simulink model "validazione_modello"  (R2021a)
settings: Solver=FixedStepAuto  StartTime=0.0  StopTime=10.0  FixedStep=Tc  RelTol=1e-3
values from neighbouring files (symbols this model uses):
  a1 = a(2)    [esercizio2.m]
  a2 = a(3)    [esercizio2.m]
  a3 = a(4)    [esercizio2.m]
  a4 = a(5)    [esercizio2.m]
  b0 = b(1)    [esercizio2.m]
  b1 = b(2)    [esercizio2.m]
  b2 = b(3)    [esercizio2.m]
  b3 = b(4)    [esercizio2.m]
  b4 = b(5)    [esercizio2.m]
settings Model: Creator=Giorgio  LastModifiedBy=Giorgio

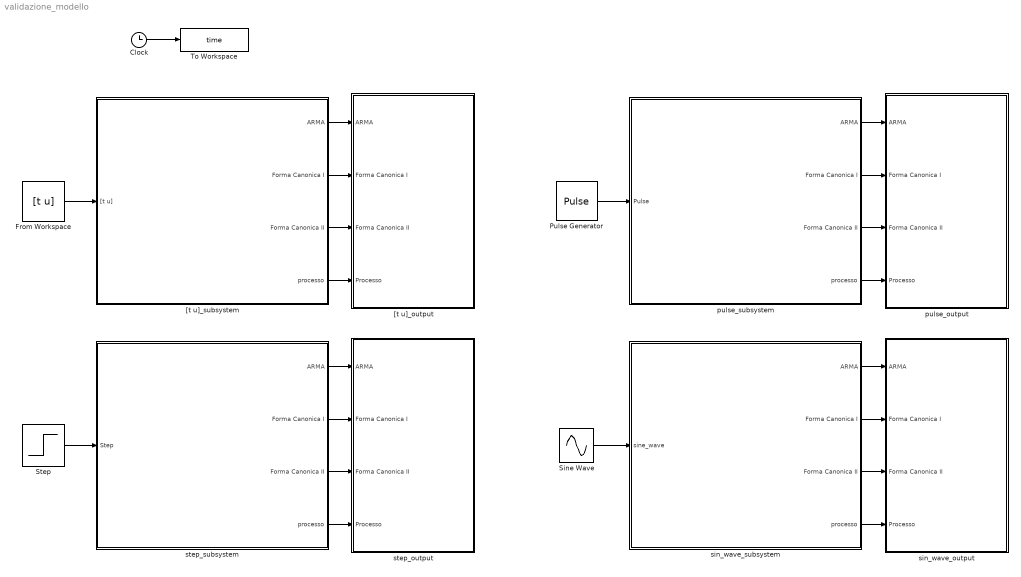
== system validazione_modello ==
  Clock : Clock
  From Workspace : FromWorkspace  VariableName=[t u]
  Pulse Generator : DiscretePulseGenerator  PulseType=Time based  Period=1  PulseWidth=50
  Sine Wave : Sin  Amplitude=0.5  Frequency=4  SampleTime=0
  Step : Step  Time=0  SampleTime=0
  To Workspace : ToWorkspace  VariableName=time  SampleTime=-1
      settings: Save2DSignal=2-D array (concatenate along first dimension)
  "[t u]_output" : Subsystem
  "[t u]_subsystem" : Subsystem
  pulse_output : Subsystem
  pulse_subsystem : Subsystem
  sin_wave_output : Subsystem
  sin_wave_subsystem : Subsystem
  step_output : Subsystem
  step_subsystem : Subsystem
  wires:
  From Workspace/1 -> "[t u]_subsystem"/1("[t u]")
  "[t u]_subsystem"/1(ARMA) -> "[t u]_output"/1(ARMA)
  "[t u]_subsystem"/2(Forma Canonica I) -> "[t u]_output"/2(Forma Canonica I)
  "[t u]_subsystem"/3(Forma Canonica II) -> "[t u]_output"/3(Forma Canonica II)
  "[t u]_subsystem"/4(processo) -> "[t u]_output"/4(Processo)
  step_subsystem/3(Forma Canonica II) -> step_output/3(Forma Canonica II)
  step_subsystem/4(processo) -> step_output/4(Processo)
  Step/1 -> step_subsystem/1(Step)
  step_subsystem/2(Forma Canonica I) -> step_output/2(Forma Canonica I)
  step_subsystem/1(ARMA) -> step_output/1(ARMA)
  pulse_subsystem/1(ARMA) -> pulse_output/1(ARMA)
  pulse_subsystem/3(Forma Canonica II) -> pulse_output/3(Forma Canonica II)
  pulse_subsystem/4(processo) -> pulse_output/4(Processo)
  pulse_subsystem/2(Forma Canonica I) -> pulse_output/2(Forma Canonica I)
  Pulse Generator/1 -> pulse_subsystem/1(Pulse)
  Clock/1 -> To Workspace/1
  sin_wave_subsystem/3(Forma Canonica II) -> sin_wave_output/3(Forma Canonica II)
  Sine Wave/1 -> sin_wave_subsystem/1(sine_wave)
  sin_wave_subsystem/2(Forma Canonica I) -> sin_wave_output/2(Forma Canonica I)
  sin_wave_subsystem/4(processo) -> sin_wave_output/4(Processo)
  sin_wave_subsystem/1(ARMA) -> sin_wave_output/1(ARMA)

== system validazione_modello/[t u]_output ==
  ARMA : Inport
  Forma Canonica I : Inport  Port=2
  Forma Canonica II : Inport  Port=3
  Processo : Inport  Port=4
  Mux : Mux
  To Workspace12 : ToWorkspace  VariableName=tu_output  SampleTime=-1
      settings: Save2DSignal=2-D array (concatenate along first dimension)
  wires:
  Mux/1 -> To Workspace12/1
  Processo/1 -> Mux/4
  Forma Canonica II/1 -> Mux/3
  ARMA/1 -> Mux/1
  Forma Canonica I/1 -> Mux/2

== system validazione_modello/[t u]_subsystem ==
  "[t u]" : Inport
  Forma Canonica di tipo I : Subsystem
  Forma Canonica di tipo II : Subsystem
  Processo : MATLABSystem  System=linSysObj  SimulateUsing=Interpreted execution
      mask Type: linSysObj
      mask Display:
      | disp('Black box');
      | port_label('input',1,'u');
      | port_label('output',1,'y');
  modello ARMA : Subsystem
  ARMA : Outport
  Forma Canonica I : Outport  Port=2
  Forma Canonica II : Outport  Port=3
  processo : Outport  Port=4
  wires:
  "[t u]"/1 -> Processo/1, Forma Canonica di tipo II/1(u(k)), Forma Canonica di tipo I/1(u(k)), modello ARMA/1(u(k))
  modello ARMA/1(y(k)) -> ARMA/1
  Forma Canonica di tipo I/1(y(k)) -> Forma Canonica I/1
  Forma Canonica di tipo II/1(y(k)) -> Forma Canonica II/1
  Processo/1 -> processo/1

== system validazione_modello/pulse_output ==
  ARMA : Inport
  Forma Canonica I : Inport  Port=2
  Forma Canonica II : Inport  Port=3
  Processo : Inport  Port=4
  Mux : Mux
  To Workspace : ToWorkspace  VariableName=pulse_processo  SampleTime=-1
      settings: Save2DSignal=2-D array (concatenate along first dimension)
  To Workspace1 : ToWorkspace  VariableName=pulse_ARMA  SampleTime=-1
      settings: Save2DSignal=2-D array (concatenate along first dimension)
  To Workspace12 : ToWorkspace  VariableName=pulse_output  SampleTime=-1
      settings: Save2DSignal=2-D array (concatenate along first dimension)
  wires:
  Mux/1 -> To Workspace12/1
  Processo/1 -> To Workspace/1, Mux/4
  Forma Canonica II/1 -> Mux/3
  ARMA/1 -> To Workspace1/1, Mux/1
  Forma Canonica I/1 -> Mux/2

== system validazione_modello/pulse_subsystem ==
  Pulse : Inport
  Forma Canonica di tipo I : Subsystem
  Forma Canonica di tipo II : Subsystem
  Processo : MATLABSystem  System=linSysObj  SimulateUsing=Interpreted execution
      mask Type: linSysObj
      mask Display:
      | disp('Black box');
      | port_label('input',1,'u');
      | port_label('output',1,'y');
  modello ARMA : Subsystem
  ARMA : Outport
  Forma Canonica I : Outport  Port=2
  Forma Canonica II : Outport  Port=3
  processo : Outport  Port=4
  wires:
  Pulse/1 -> Processo/1, Forma Canonica di tipo II/1(u(k)), Forma Canonica di tipo I/1(u(k)), modello ARMA/1(u(k))
  modello ARMA/1(y(k)) -> ARMA/1
  Forma Canonica di tipo I/1(y(k)) -> Forma Canonica I/1
  Forma Canonica di tipo II/1(y(k)) -> Forma Canonica II/1
  Processo/1 -> processo/1

== system validazione_modello/sin_wave_output ==
  ARMA : Inport
  Forma Canonica I : Inport  Port=2
  Forma Canonica II : Inport  Port=3
  Processo : Inport  Port=4
  Mux : Mux
  To Workspace : ToWorkspace  VariableName=sine_wave_ARMA  SampleTime=-1
      settings: Save2DSignal=2-D array (concatenate along first dimension)
  To Workspace1 : ToWorkspace  VariableName=sine_wave_processo  SampleTime=-1
      settings: Save2DSignal=2-D array (concatenate along first dimension)
  To Workspace12 : ToWorkspace  VariableName=sine_wave_output  SampleTime=-1
      settings: Save2DSignal=2-D array (concatenate along first dimension)
  wires:
  Mux/1 -> To Workspace12/1
  Processo/1 -> To Workspace1/1, Mux/4
  Forma Canonica II/1 -> Mux/3
  ARMA/1 -> To Workspace/1, Mux/1
  Forma Canonica I/1 -> Mux/2

== system validazione_modello/sin_wave_subsystem ==
  sine_wave : Inport
  Forma Canonica di tipo I : Subsystem
  Forma Canonica di tipo II : Subsystem
  Processo : MATLABSystem  System=linSysObj  SimulateUsing=Interpreted execution
      mask Type: linSysObj
      mask Display:
      | disp('Black box');
      | port_label('input',1,'u');
      | port_label('output',1,'y');
  modello ARMA : Subsystem
  ARMA : Outport
  Forma Canonica I : Outport  Port=2
  Forma Canonica II : Outport  Port=3
  processo : Outport  Port=4
  wires:
  sine_wave/1 -> Processo/1, Forma Canonica di tipo II/1(u(k)), Forma Canonica di tipo I/1(u(k)), modello ARMA/1(u(k))
  modello ARMA/1(y(k)) -> ARMA/1
  Forma Canonica di tipo I/1(y(k)) -> Forma Canonica I/1
  Forma Canonica di tipo II/1(y(k)) -> Forma Canonica II/1
  Processo/1 -> processo/1

== system validazione_modello/step_output ==
  ARMA : Inport
  Forma Canonica I : Inport  Port=2
  Forma Canonica II : Inport  Port=3
  Processo : Inport  Port=4
  Mux : Mux
  To Workspace : ToWorkspace  VariableName=step_processo  SampleTime=-1
      settings: Save2DSignal=2-D array (concatenate along first dimension)
  To Workspace1 : ToWorkspace  VariableName=step_ARMA  SampleTime=-1
      settings: Save2DSignal=2-D array (concatenate along first dimension)
  To Workspace12 : ToWorkspace  VariableName=step_output  SampleTime=-1
      settings: Save2DSignal=2-D array (concatenate along first dimension)
  wires:
  Mux/1 -> To Workspace12/1
  Processo/1 -> Mux/4, To Workspace/1
  Forma Canonica II/1 -> Mux/3
  ARMA/1 -> Mux/1, To Workspace1/1
  Forma Canonica I/1 -> Mux/2

== system validazione_modello/step_subsystem ==
  Step : Inport
  Forma Canonica di tipo I : Subsystem
  Forma Canonica di tipo II : Subsystem
  Processo : MATLABSystem  System=linSysObj  SimulateUsing=Interpreted execution
      mask Type: linSysObj
      mask Display:
      | disp('Black box');
      | port_label('input',1,'u');
      | port_label('output',1,'y');
  modello ARMA : Subsystem
  ARMA : Outport
  Forma Canonica I : Outport  Port=2
  Forma Canonica II : Outport  Port=3
  processo : Outport  Port=4
  wires:
  Step/1 -> Processo/1, Forma Canonica di tipo II/1(u(k)), Forma Canonica di tipo I/1(u(k)), modello ARMA/1(u(k))
  modello ARMA/1(y(k)) -> ARMA/1
  Forma Canonica di tipo I/1(y(k)) -> Forma Canonica I/1
  Forma Canonica di tipo II/1(y(k)) -> Forma Canonica II/1
  Processo/1 -> processo/1

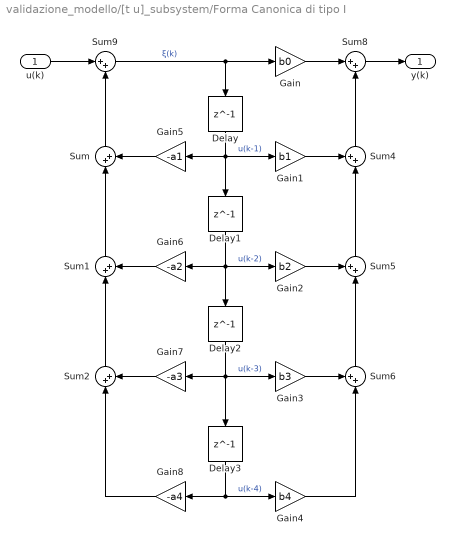
== system validazione_modello/[t u]_subsystem/Forma Canonica di tipo I ==
  u(k) : Inport
  Delay{,1..3} (4 alike) : Delay  DelayLength=1
  Gain : Gain  Gain=b0
  Gain1 : Gain  Gain=b1
  Gain2 : Gain  Gain=b2
  Gain3 : Gain  Gain=b3
  Gain4 : Gain  Gain=b4
  Gain5 : Gain  Gain=-a1
  Gain6 : Gain  Gain=-a2
  Gain7 : Gain  Gain=-a3
  Gain8 : Gain  Gain=-a4
  Sum{,1..2,8..9} (5 alike) : Sum  Inputs=|++
  Sum4 : Sum  Inputs=++|
  Sum5 : Sum  Inputs=++|
  Sum6 : Sum  Inputs=++|
  y(k) : Outport
  wires:
  Sum1/1 -> Sum/1
  Sum2/1 -> Sum1/1
  Gain8/1 -> Sum2/1
  Sum8/1 -> y(k)/1
  Sum4/1 -> Sum8/2
  Sum5/1 -> Sum4/2
  Sum6/1 -> Sum5/2
  Gain4/1 -> Sum6/2
  Delay/1 -> Gain1/1, Delay1/1, Gain5/1  "u(k-1)"
  Delay1/1 -> Delay2/1, Gain6/1, Gain2/1  "u(k-2)"
  Delay2/1 -> Gain7/1, Gain3/1, Delay3/1  "u(k-3)"
  Delay3/1 -> Gain8/1, Gain4/1  "u(k-4)"
  Sum/1 -> Sum9/2
  u(k)/1 -> Sum9/1
  Sum9/1 -> Gain/1, Delay/1  "ξ(k)"
  Gain/1 -> Sum8/1
  Gain1/1 -> Sum4/1
  Gain2/1 -> Sum5/1
  Gain3/1 -> Sum6/1
  Gain5/1 -> Sum/2
  Gain6/1 -> Sum1/2
  Gain7/1 -> Sum2/2

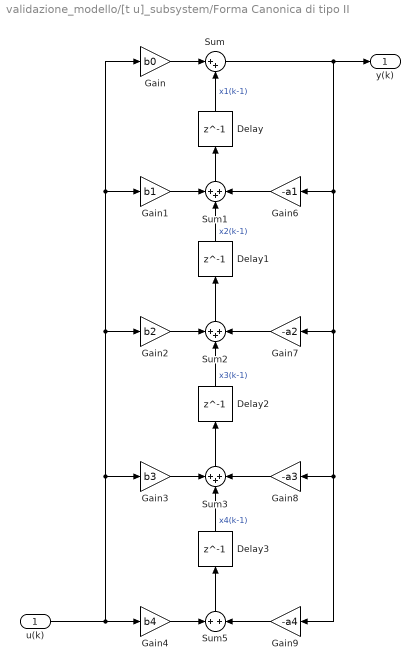
== system validazione_modello/[t u]_subsystem/Forma Canonica di tipo II ==
  u(k) : Inport
  Delay{,1..3} (4 alike) : Delay  DelayLength=1
  Gain : Gain  Gain=b0
  Gain1 : Gain  Gain=b1
  Gain2 : Gain  Gain=b2
  Gain3 : Gain  Gain=b3
  Gain4 : Gain  Gain=b4
  Gain6 : Gain  Gain=-a1
  Gain7 : Gain  Gain=-a2
  Gain8 : Gain  Gain=-a3
  Gain9 : Gain  Gain=-a4
  Sum : Sum  Inputs=|++
  Sum1 : Sum  Inputs=+++
  Sum2 : Sum  Inputs=+++
  Sum3 : Sum  Inputs=+++
  Sum5 : Sum  Inputs=+|+
  y(k) : Outport
  wires:
  u(k)/1 -> Gain4/1, Gain3/1, Gain2/1, Gain/1, Gain1/1
  Sum/1 -> Gain6/1, Gain7/1, Gain8/1, Gain9/1, y(k)/1
  Gain/1 -> Sum/1
  Sum1/1 -> Delay/1
  Sum2/1 -> Delay1/1
  Sum3/1 -> Delay2/1
  Gain1/1 -> Sum1/1
  Gain2/1 -> Sum2/1
  Gain3/1 -> Sum3/1
  Gain4/1 -> Sum5/1
  Gain8/1 -> Sum3/3
  Gain7/1 -> Sum2/3
  Gain6/1 -> Sum1/3
  Gain9/1 -> Sum5/2
  Delay/1 -> Sum/2  "x1(k-1)"
  Delay1/1 -> Sum1/2  "x2(k-1)"
  Delay2/1 -> Sum2/2  "x3(k-1)"
  Sum5/1 -> Delay3/1
  Delay3/1 -> Sum3/2  "x4(k-1)"

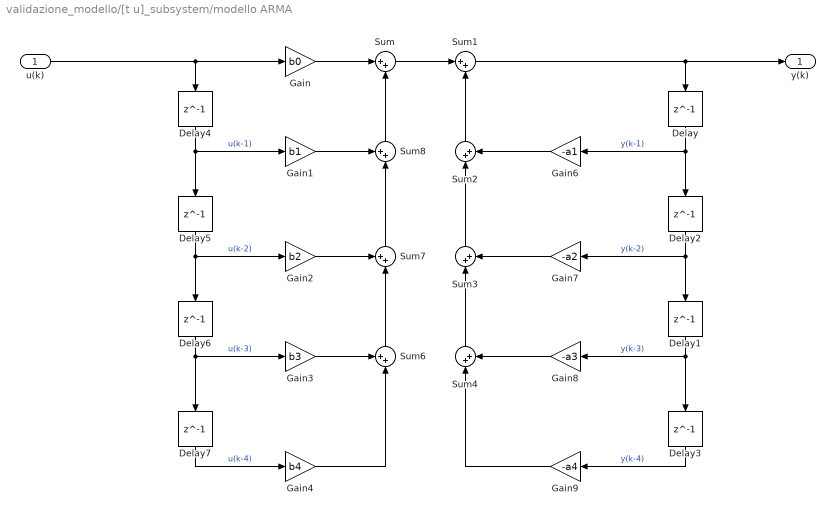
== system validazione_modello/[t u]_subsystem/modello ARMA ==
  u(k) : Inport
  Delay{,1..7} (8 alike) : Delay  DelayLength=1
  Gain : Gain  Gain=b0
  Gain1 : Gain  Gain=b1
  Gain2 : Gain  Gain=b2
  Gain3 : Gain  Gain=b3
  Gain4 : Gain  Gain=b4
  Gain6 : Gain  Gain=-a1
  Gain7 : Gain  Gain=-a2
  Gain8 : Gain  Gain=-a3
  Gain9 : Gain  Gain=-a4
  Sum{,1..4} (5 alike) : Sum  Inputs=|++
  Sum6 : Sum  Inputs=++|
  Sum7 : Sum  Inputs=++|
  Sum8 : Sum  Inputs=++|
  y(k) : Outport
  wires:
  Gain3/1 -> Sum6/1
  Gain9/1 -> Sum4/1
  Gain8/1 -> Sum4/2
  Gain4/1 -> Sum6/2
  Sum7/1 -> Sum8/2
  Sum/1 -> Sum1/1
  Gain1/1 -> Sum8/1
  Gain6/1 -> Sum2/2
  Gain7/1 -> Sum3/2
  Delay1/1 -> Delay3/1, Gain8/1  "y(k-3)"
  Gain/1 -> Sum/1
  Delay5/1 -> Delay6/1, Gain2/1  "u(k-2)"
  Sum4/1 -> Sum3/1
  Sum8/1 -> Sum/2
  Delay6/1 -> Delay7/1, Gain3/1  "u(k-3)"
  Sum2/1 -> Sum1/2
  Delay2/1 -> Delay1/1, Gain7/1  "y(k-2)"
  Delay/1 -> Delay2/1, Gain6/1  "y(k-1)"
  Sum3/1 -> Sum2/1
  Gain2/1 -> Sum7/1
  Sum1/1 -> y(k)/1, Delay/1
  Delay4/1 -> Delay5/1, Gain1/1  "u(k-1)"
  Sum6/1 -> Sum7/2
  u(k)/1 -> Gain/1, Delay4/1
  Delay7/1 -> Gain4/1  "u(k-4)"
  Delay3/1 -> Gain9/1  "y(k-4)"

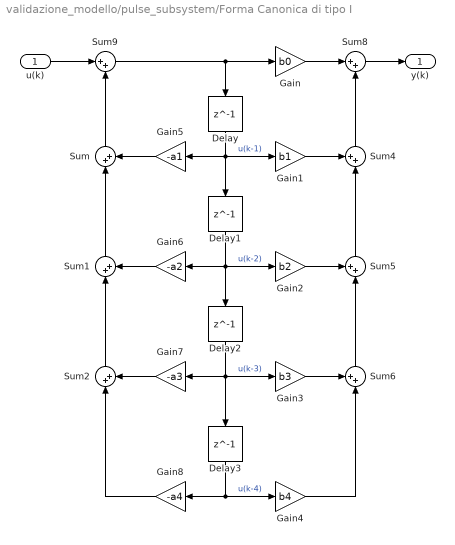
== system validazione_modello/pulse_subsystem/Forma Canonica di tipo I ==
  u(k) : Inport
  Delay{,1..3} (4 alike) : Delay  DelayLength=1
  Gain : Gain  Gain=b0
  Gain1 : Gain  Gain=b1
  Gain2 : Gain  Gain=b2
  Gain3 : Gain  Gain=b3
  Gain4 : Gain  Gain=b4
  Gain5 : Gain  Gain=-a1
  Gain6 : Gain  Gain=-a2
  Gain7 : Gain  Gain=-a3
  Gain8 : Gain  Gain=-a4
  Sum{,1..2,8..9} (5 alike) : Sum  Inputs=|++
  Sum4 : Sum  Inputs=++|
  Sum5 : Sum  Inputs=++|
  Sum6 : Sum  Inputs=++|
  y(k) : Outport
  wires:
  Sum1/1 -> Sum/1
  Sum2/1 -> Sum1/1
  Gain8/1 -> Sum2/1
  Sum8/1 -> y(k)/1
  Sum4/1 -> Sum8/2
  Sum5/1 -> Sum4/2
  Sum6/1 -> Sum5/2
  Gain4/1 -> Sum6/2
  Delay/1 -> Gain1/1, Delay1/1, Gain5/1  "u(k-1)"
  Delay1/1 -> Delay2/1, Gain6/1, Gain2/1  "u(k-2)"
  Delay2/1 -> Gain7/1, Gain3/1, Delay3/1  "u(k-3)"
  Delay3/1 -> Gain8/1, Gain4/1  "u(k-4)"
  Sum/1 -> Sum9/2
  u(k)/1 -> Sum9/1
  Sum9/1 -> Gain/1, Delay/1
  Gain/1 -> Sum8/1
  Gain1/1 -> Sum4/1
  Gain2/1 -> Sum5/1
  Gain3/1 -> Sum6/1
  Gain5/1 -> Sum/2
  Gain6/1 -> Sum1/2
  Gain7/1 -> Sum2/2

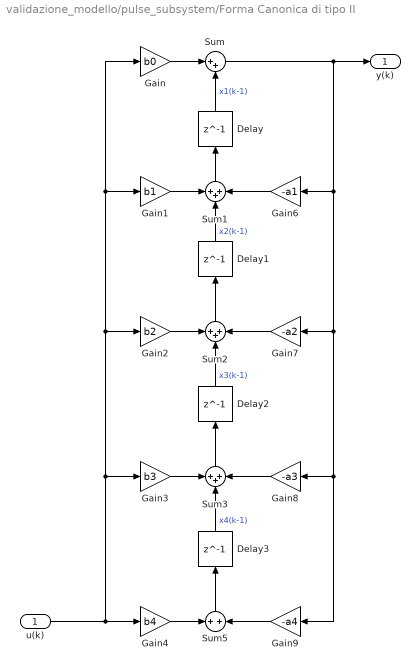
== system validazione_modello/pulse_subsystem/Forma Canonica di tipo II ==
  u(k) : Inport
  Delay{,1..3} (4 alike) : Delay  DelayLength=1
  Gain : Gain  Gain=b0
  Gain1 : Gain  Gain=b1
  Gain2 : Gain  Gain=b2
  Gain3 : Gain  Gain=b3
  Gain4 : Gain  Gain=b4
  Gain6 : Gain  Gain=-a1
  Gain7 : Gain  Gain=-a2
  Gain8 : Gain  Gain=-a3
  Gain9 : Gain  Gain=-a4
  Sum : Sum  Inputs=|++
  Sum1 : Sum  Inputs=+++
  Sum2 : Sum  Inputs=+++
  Sum3 : Sum  Inputs=+++
  Sum5 : Sum  Inputs=+|+
  y(k) : Outport
  wires:
  u(k)/1 -> Gain4/1, Gain3/1, Gain2/1, Gain/1, Gain1/1
  Sum/1 -> Gain6/1, Gain7/1, Gain8/1, Gain9/1, y(k)/1
  Gain/1 -> Sum/1
  Sum1/1 -> Delay/1
  Sum2/1 -> Delay1/1
  Sum3/1 -> Delay2/1
  Gain1/1 -> Sum1/1
  Gain2/1 -> Sum2/1
  Gain3/1 -> Sum3/1
  Gain4/1 -> Sum5/1
  Gain8/1 -> Sum3/3
  Gain7/1 -> Sum2/3
  Gain6/1 -> Sum1/3
  Gain9/1 -> Sum5/2
  Delay/1 -> Sum/2  "x1(k-1)"
  Delay1/1 -> Sum1/2  "x2(k-1)"
  Delay2/1 -> Sum2/2  "x3(k-1)"
  Sum5/1 -> Delay3/1
  Delay3/1 -> Sum3/2  "x4(k-1)"

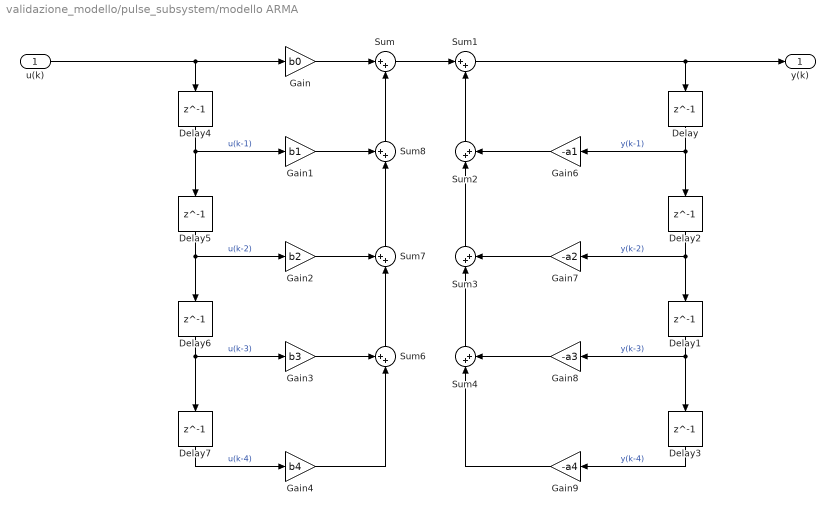
== system validazione_modello/pulse_subsystem/modello ARMA ==
  u(k) : Inport
  Delay{,1..7} (8 alike) : Delay  DelayLength=1
  Gain : Gain  Gain=b0
  Gain1 : Gain  Gain=b1
  Gain2 : Gain  Gain=b2
  Gain3 : Gain  Gain=b3
  Gain4 : Gain  Gain=b4
  Gain6 : Gain  Gain=-a1
  Gain7 : Gain  Gain=-a2
  Gain8 : Gain  Gain=-a3
  Gain9 : Gain  Gain=-a4
  Sum{,1..4} (5 alike) : Sum  Inputs=|++
  Sum6 : Sum  Inputs=++|
  Sum7 : Sum  Inputs=++|
  Sum8 : Sum  Inputs=++|
  y(k) : Outport
  wires:
  Gain3/1 -> Sum6/1
  Gain9/1 -> Sum4/1
  Gain8/1 -> Sum4/2
  Gain4/1 -> Sum6/2
  Sum7/1 -> Sum8/2
  Sum/1 -> Sum1/1
  Gain1/1 -> Sum8/1
  Gain6/1 -> Sum2/2
  Gain7/1 -> Sum3/2
  Delay1/1 -> Delay3/1, Gain8/1  "y(k-3)"
  Gain/1 -> Sum/1
  Delay5/1 -> Delay6/1, Gain2/1  "u(k-2)"
  Sum4/1 -> Sum3/1
  Sum8/1 -> Sum/2
  Delay6/1 -> Delay7/1, Gain3/1  "u(k-3)"
  Sum2/1 -> Sum1/2
  Delay2/1 -> Delay1/1, Gain7/1  "y(k-2)"
  Delay/1 -> Delay2/1, Gain6/1  "y(k-1)"
  Sum3/1 -> Sum2/1
  Gain2/1 -> Sum7/1
  Sum1/1 -> y(k)/1, Delay/1
  Delay4/1 -> Delay5/1, Gain1/1  "u(k-1)"
  Sum6/1 -> Sum7/2
  u(k)/1 -> Gain/1, Delay4/1
  Delay7/1 -> Gain4/1  "u(k-4)"
  Delay3/1 -> Gain9/1  "y(k-4)"

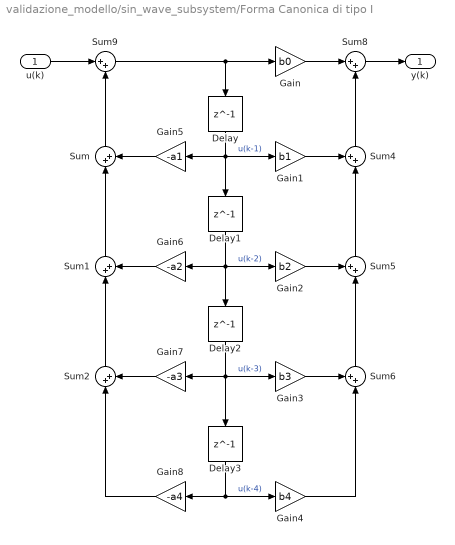
== system validazione_modello/sin_wave_subsystem/Forma Canonica di tipo I ==
  u(k) : Inport
  Delay{,1..3} (4 alike) : Delay  DelayLength=1
  Gain : Gain  Gain=b0
  Gain1 : Gain  Gain=b1
  Gain2 : Gain  Gain=b2
  Gain3 : Gain  Gain=b3
  Gain4 : Gain  Gain=b4
  Gain5 : Gain  Gain=-a1
  Gain6 : Gain  Gain=-a2
  Gain7 : Gain  Gain=-a3
  Gain8 : Gain  Gain=-a4
  Sum{,1..2,8..9} (5 alike) : Sum  Inputs=|++
  Sum4 : Sum  Inputs=++|
  Sum5 : Sum  Inputs=++|
  Sum6 : Sum  Inputs=++|
  y(k) : Outport
  wires:
  Sum1/1 -> Sum/1
  Sum2/1 -> Sum1/1
  Gain8/1 -> Sum2/1
  Sum8/1 -> y(k)/1
  Sum4/1 -> Sum8/2
  Sum5/1 -> Sum4/2
  Sum6/1 -> Sum5/2
  Gain4/1 -> Sum6/2
  Delay/1 -> Gain1/1, Delay1/1, Gain5/1  "u(k-1)"
  Delay1/1 -> Delay2/1, Gain6/1, Gain2/1  "u(k-2)"
  Delay2/1 -> Gain7/1, Gain3/1, Delay3/1  "u(k-3)"
  Delay3/1 -> Gain8/1, Gain4/1  "u(k-4)"
  Sum/1 -> Sum9/2
  u(k)/1 -> Sum9/1
  Sum9/1 -> Gain/1, Delay/1
  Gain/1 -> Sum8/1
  Gain1/1 -> Sum4/1
  Gain2/1 -> Sum5/1
  Gain3/1 -> Sum6/1
  Gain5/1 -> Sum/2
  Gain6/1 -> Sum1/2
  Gain7/1 -> Sum2/2

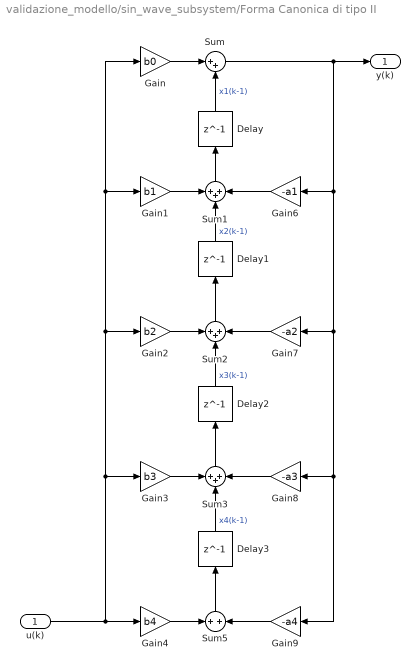
== system validazione_modello/sin_wave_subsystem/Forma Canonica di tipo II ==
  u(k) : Inport
  Delay{,1..3} (4 alike) : Delay  DelayLength=1
  Gain : Gain  Gain=b0
  Gain1 : Gain  Gain=b1
  Gain2 : Gain  Gain=b2
  Gain3 : Gain  Gain=b3
  Gain4 : Gain  Gain=b4
  Gain6 : Gain  Gain=-a1
  Gain7 : Gain  Gain=-a2
  Gain8 : Gain  Gain=-a3
  Gain9 : Gain  Gain=-a4
  Sum : Sum  Inputs=|++
  Sum1 : Sum  Inputs=+++
  Sum2 : Sum  Inputs=+++
  Sum3 : Sum  Inputs=+++
  Sum5 : Sum  Inputs=+|+
  y(k) : Outport
  wires:
  u(k)/1 -> Gain4/1, Gain3/1, Gain2/1, Gain/1, Gain1/1
  Sum/1 -> Gain6/1, Gain7/1, Gain8/1, Gain9/1, y(k)/1
  Gain/1 -> Sum/1
  Sum1/1 -> Delay/1
  Sum2/1 -> Delay1/1
  Sum3/1 -> Delay2/1
  Gain1/1 -> Sum1/1
  Gain2/1 -> Sum2/1
  Gain3/1 -> Sum3/1
  Gain4/1 -> Sum5/1
  Gain8/1 -> Sum3/3
  Gain7/1 -> Sum2/3
  Gain6/1 -> Sum1/3
  Gain9/1 -> Sum5/2
  Delay/1 -> Sum/2  "x1(k-1)"
  Delay1/1 -> Sum1/2  "x2(k-1)"
  Delay2/1 -> Sum2/2  "x3(k-1)"
  Sum5/1 -> Delay3/1
  Delay3/1 -> Sum3/2  "x4(k-1)"

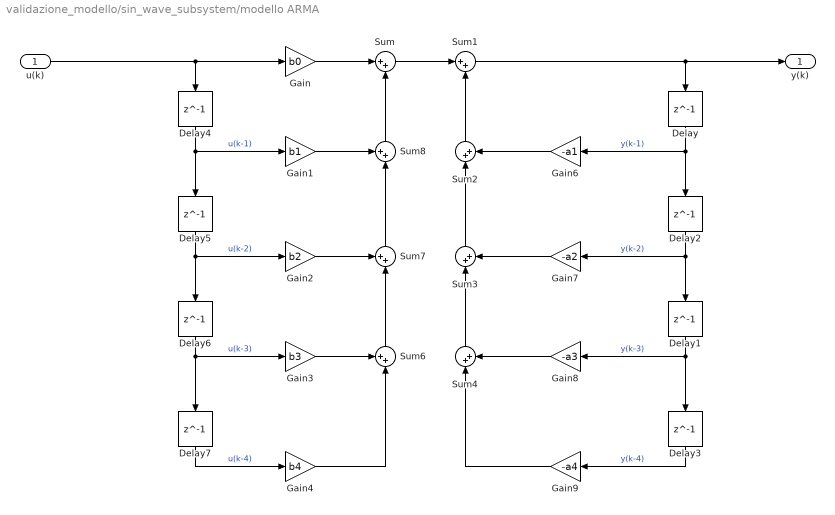
== system validazione_modello/sin_wave_subsystem/modello ARMA ==
  u(k) : Inport
  Delay{,1..7} (8 alike) : Delay  DelayLength=1
  Gain : Gain  Gain=b0
  Gain1 : Gain  Gain=b1
  Gain2 : Gain  Gain=b2
  Gain3 : Gain  Gain=b3
  Gain4 : Gain  Gain=b4
  Gain6 : Gain  Gain=-a1
  Gain7 : Gain  Gain=-a2
  Gain8 : Gain  Gain=-a3
  Gain9 : Gain  Gain=-a4
  Sum{,1..4} (5 alike) : Sum  Inputs=|++
  Sum6 : Sum  Inputs=++|
  Sum7 : Sum  Inputs=++|
  Sum8 : Sum  Inputs=++|
  y(k) : Outport
  wires:
  Gain3/1 -> Sum6/1
  Gain9/1 -> Sum4/1
  Gain8/1 -> Sum4/2
  Gain4/1 -> Sum6/2
  Sum7/1 -> Sum8/2
  Sum/1 -> Sum1/1
  Gain1/1 -> Sum8/1
  Gain6/1 -> Sum2/2
  Gain7/1 -> Sum3/2
  Delay1/1 -> Delay3/1, Gain8/1  "y(k-3)"
  Gain/1 -> Sum/1
  Delay5/1 -> Delay6/1, Gain2/1  "u(k-2)"
  Sum4/1 -> Sum3/1
  Sum8/1 -> Sum/2
  Delay6/1 -> Delay7/1, Gain3/1  "u(k-3)"
  Sum2/1 -> Sum1/2
  Delay2/1 -> Delay1/1, Gain7/1  "y(k-2)"
  Delay/1 -> Delay2/1, Gain6/1  "y(k-1)"
  Sum3/1 -> Sum2/1
  Gain2/1 -> Sum7/1
  Sum1/1 -> y(k)/1, Delay/1
  Delay4/1 -> Delay5/1, Gain1/1  "u(k-1)"
  Sum6/1 -> Sum7/2
  u(k)/1 -> Gain/1, Delay4/1
  Delay7/1 -> Gain4/1  "u(k-4)"
  Delay3/1 -> Gain9/1  "y(k-4)"

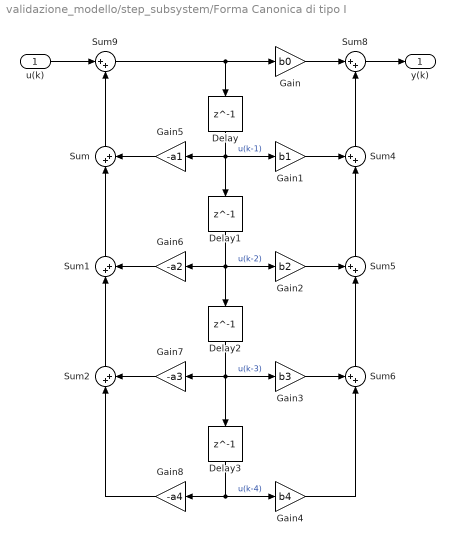
== system validazione_modello/step_subsystem/Forma Canonica di tipo I ==
  u(k) : Inport
  Delay{,1..3} (4 alike) : Delay  DelayLength=1
  Gain : Gain  Gain=b0
  Gain1 : Gain  Gain=b1
  Gain2 : Gain  Gain=b2
  Gain3 : Gain  Gain=b3
  Gain4 : Gain  Gain=b4
  Gain5 : Gain  Gain=-a1
  Gain6 : Gain  Gain=-a2
  Gain7 : Gain  Gain=-a3
  Gain8 : Gain  Gain=-a4
  Sum{,1..2,8..9} (5 alike) : Sum  Inputs=|++
  Sum4 : Sum  Inputs=++|
  Sum5 : Sum  Inputs=++|
  Sum6 : Sum  Inputs=++|
  y(k) : Outport
  wires:
  Sum1/1 -> Sum/1
  Sum2/1 -> Sum1/1
  Gain8/1 -> Sum2/1
  Sum8/1 -> y(k)/1
  Sum4/1 -> Sum8/2
  Sum5/1 -> Sum4/2
  Sum6/1 -> Sum5/2
  Gain4/1 -> Sum6/2
  Delay/1 -> Gain1/1, Delay1/1, Gain5/1  "u(k-1)"
  Delay1/1 -> Delay2/1, Gain6/1, Gain2/1  "u(k-2)"
  Delay2/1 -> Gain7/1, Gain3/1, Delay3/1  "u(k-3)"
  Delay3/1 -> Gain8/1, Gain4/1  "u(k-4)"
  Sum/1 -> Sum9/2
  u(k)/1 -> Sum9/1
  Sum9/1 -> Gain/1, Delay/1
  Gain/1 -> Sum8/1
  Gain1/1 -> Sum4/1
  Gain2/1 -> Sum5/1
  Gain3/1 -> Sum6/1
  Gain5/1 -> Sum/2
  Gain6/1 -> Sum1/2
  Gain7/1 -> Sum2/2

== system validazione_modello/step_subsystem/Forma Canonica di tipo II ==
  u(k) : Inport
  Delay{,1..3} (4 alike) : Delay  DelayLength=1
  Gain : Gain  Gain=b0
  Gain1 : Gain  Gain=b1
  Gain2 : Gain  Gain=b2
  Gain3 : Gain  Gain=b3
  Gain4 : Gain  Gain=b4
  Gain6 : Gain  Gain=-a1
  Gain7 : Gain  Gain=-a2
  Gain8 : Gain  Gain=-a3
  Gain9 : Gain  Gain=-a4
  Sum : Sum  Inputs=|++
  Sum1 : Sum  Inputs=+++
  Sum2 : Sum  Inputs=+++
  Sum3 : Sum  Inputs=+++
  Sum5 : Sum  Inputs=+|+
  y(k) : Outport
  wires:
  u(k)/1 -> Gain4/1, Gain3/1, Gain2/1, Gain/1, Gain1/1
  Sum/1 -> Gain6/1, Gain7/1, Gain8/1, Gain9/1, y(k)/1
  Gain/1 -> Sum/1
  Sum1/1 -> Delay/1
  Sum2/1 -> Delay1/1
  Sum3/1 -> Delay2/1
  Gain1/1 -> Sum1/1
  Gain2/1 -> Sum2/1
  Gain3/1 -> Sum3/1
  Gain4/1 -> Sum5/1
  Gain8/1 -> Sum3/3
  Gain7/1 -> Sum2/3
  Gain6/1 -> Sum1/3
  Gain9/1 -> Sum5/2
  Delay/1 -> Sum/2  "x1(k-1)"
  Delay1/1 -> Sum1/2  "x2(k-1)"
  Delay2/1 -> Sum2/2  "x3(k-1)"
  Sum5/1 -> Delay3/1
  Delay3/1 -> Sum3/2  "x4(k-1)"

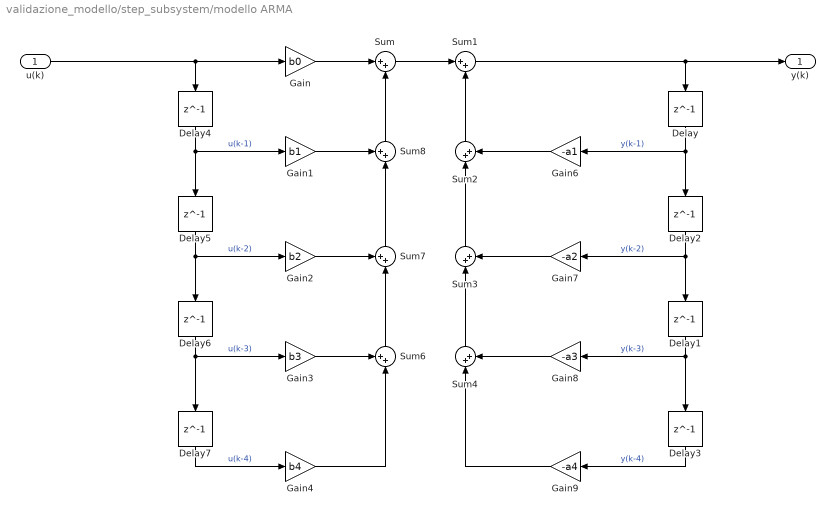
== system validazione_modello/step_subsystem/modello ARMA ==
  u(k) : Inport
  Delay{,1..7} (8 alike) : Delay  DelayLength=1
  Gain : Gain  Gain=b0
  Gain1 : Gain  Gain=b1
  Gain2 : Gain  Gain=b2
  Gain3 : Gain  Gain=b3
  Gain4 : Gain  Gain=b4
  Gain6 : Gain  Gain=-a1
  Gain7 : Gain  Gain=-a2
  Gain8 : Gain  Gain=-a3
  Gain9 : Gain  Gain=-a4
  Sum{,1..4} (5 alike) : Sum  Inputs=|++
  Sum6 : Sum  Inputs=++|
  Sum7 : Sum  Inputs=++|
  Sum8 : Sum  Inputs=++|
  y(k) : Outport
  wires:
  Gain3/1 -> Sum6/1
  Gain9/1 -> Sum4/1
  Gain8/1 -> Sum4/2
  Gain4/1 -> Sum6/2
  Sum7/1 -> Sum8/2
  Sum/1 -> Sum1/1
  Gain1/1 -> Sum8/1
  Gain6/1 -> Sum2/2
  Gain7/1 -> Sum3/2
  Delay1/1 -> Delay3/1, Gain8/1  "y(k-3)"
  Gain/1 -> Sum/1
  Delay5/1 -> Delay6/1, Gain2/1  "u(k-2)"
  Sum4/1 -> Sum3/1
  Sum8/1 -> Sum/2
  Delay6/1 -> Delay7/1, Gain3/1  "u(k-3)"
  Sum2/1 -> Sum1/2
  Delay2/1 -> Delay1/1, Gain7/1  "y(k-2)"
  Delay/1 -> Delay2/1, Gain6/1  "y(k-1)"
  Sum3/1 -> Sum2/1
  Gain2/1 -> Sum7/1
  Sum1/1 -> y(k)/1, Delay/1
  Delay4/1 -> Delay5/1, Gain1/1  "u(k-1)"
  Sum6/1 -> Sum7/2
  u(k)/1 -> Gain/1, Delay4/1
  Delay7/1 -> Gain4/1  "u(k-4)"
  Delay3/1 -> Gain9/1  "y(k-4)"
